simulink model "c_citation"  (R2020a)
settings: Solver=ode5  StartTime=0.0  StopTime=inf  FixedStep=0.01  RelTol=1e-3
InitFcn:
  | load('simulation_parameters');
values from neighbouring files (symbols this model uses):
  chord = 1.991    [citdata.mat]
  cv1 = 20000    [gear_params.m]
  cv2 = cv1    (= 20000)    [gear_params.m]
  cv3 = 4000    [gear_params.m]
  cv4 = 20000    [gear_params.m]
  deltagmax1 = 0.25    [gear_params.m]
  deltagmax2 = deltagmax1    (= 0.25)    [gear_params.m]
  deltagmax3 = 0.24    [gear_params.m]
  deltagmax4 = 0.02    [gear_params.m]
  ealphag = [0  0.2618  0.6981; 1  1.3  0.8]    [citdata.mat]
  ealphas = [0  0.2618  0.6981; 0.157  0.157  0.175]    [citdata.mat]
  g0 = 9.80665    [ac_genrl.mat]
  hDME = 0    [ac_genrl.mat]
  hGS = 0    [ac_genrl.mat]
  kt1 = 525020    [gear_params.m]
  kt2 = kt1    (= 525020)    [gear_params.m]
  kt3 = 457050    [gear_params.m]
  lh = 5.53    [citdata.mat]
  matbuaf = [0  -0.1745  0.4363; 0  -0.1  -0.1; 0.6981  -0.1  -0.1]    [citdata.mat]
  matdaf = [0 0 0.2618 0.6981 0.734842105263 0.771584210526 0.808326315789 0.845068421053 0.881810526316 0.918552631579 0.955294736842 0.992036842105 ... (529 elements, 23x23)]    [citdata.mat]
  matdam = [0 0.05 0.15 0.25 0.35 0.45 0.55 0.65 0.75 0.803571428571 0.857142857143 0.910714285714 ... (529 elements, 23x23)]    [citdata.mat]
  matdbbf = [0 0 0.6981 0.74464 0.79118 0.83772 0.88426 0.9308 0.97734 1.02388 1.07042 1.11696 ... (324 elements, 18x18)]    [citdata.mat]
  matdeaf = [0 0 0.2618 0.6981 0.734842105263 0.771584210526 0.808326315789 0.845068421053 0.881810526316 0.918552631579 0.955294736842 0.992036842105 ... (529 elements, 23x23)]    [citdata.mat]
  matdgaf = [0 0 0.2618 0.6981 -0.1745 -0.0175 -0.008 -0.009 0.4363 -0.0175 -0.008 -0.009 ... (16 elements, 4x4)]    [citdata.mat]
  matdqaf = [0 0 0.2618 0.6981 0.734842105263 0.771584210526 0.808326315789 0.845068421053 0.881810526316 0.918552631579 0.955294736842 0.992036842105 ... (529 elements, 23x23)]    [citdata.mat]
  matduaf = [0 0 0.2618 0.6981 0.734842105263 0.771584210526 0.808326315789 0.845068421053 0.881810526316 0.918552631579 0.955294736842 0.992036842105 ... (529 elements, 23x23)]    [citdata.mat]
  matdwaw = [0 0 0.1745 0.3491 0.5236 0.6458 1.2916 -0.1745 0 0.0018 0.0046 0.0088 ... (49 elements, 7x7)]    [citdata.mat]
  matedhr = [0 1 1 0.71 2 0.51 3 0.34 5 0.12 7.5 0.03 ... (20 elements, 2x10)]    [citdata.mat]
  mateif = [0  0.2618  0.6981; 0  -0.075  -0.075]    [citdata.mat]
  matelhr = [0 1 1 0.95 2 0.91 3 0.84 5 0.71 7.5 0.35 ... (20 elements, 2x10)]    [citdata.mat]
  matemhr = [0 1 1 0.9 2 0.8 3 0.7 5 0.5 7.5 0.25 ... (20 elements, 2x10)]    [citdata.mat]
  matemv1 = [0  90  100; 0  1  1]    [citdata.mat]
  matemv2 = [20  75  90; 0  1  1]    [citdata.mat]
  matemve = [0  90  100; 0  1  1]    [citdata.mat]
  matetam = [0  -0.1745  0.4363; 0  -0.04  -0.04; 1  -0.04  -0.04]    [citdata.mat]
  mateuaf = [0 0 0.6981 0.733005 0.76791 0.802815 0.83772 0.872625 0.90753 0.942435 0.97734 1.012245 ... (529 elements, 23x23)]    [citdata.mat]
  matfaaf = [0 0 0.2618 0.6981 0.734842105263 0.771584210526 0.808326315789 0.845068421053 0.881810526316 0.918552631579 0.955294736842 0.992036842105 ... (529 elements, 23x23)]    [citdata.mat]
  matfaxl = [0.15  0.35; 1  1]    [citdata.mat]
  matibaf = [0 0 0.2618 0.6981 -0.2 -0.119 -0.117 -0.108 0.3 -0.059 -0.052 -0.038 ... (16 elements, 4x4)]    [citdata.mat]
  matibb = [0 0 0.2618 1.571 3.142 -0.2 0 0 0.074 0.124 0 0 ... (50 elements, 5x10)]    [citdata.mat]
  matibmh = [0 0 15000 17142.8571429 19285.7142857 21428.5714286 23571.4285714 25714.2857143 27857.1428571 30000 0 0 ... (100 elements, 10x10)]    [citdata.mat]
  matipaf = [0  -0.1745  0.4363; 0  -0.44  -0.44; 0.6981  -0.44  -0.44]    [citdata.mat]
  matipmh = [0 0 15000 17142.8571429 19285.7142857 21428.5714286 23571.4285714 25714.2857143 27857.1428571 30000 0 0 ... (100 elements, 10x10)]    [citdata.mat]
  matiraf = [0 0 0.2618 0.6981 -0.2 0.05 -0.03 0.01 0.3 0.3 0.37 0.41 ... (16 elements, 4x4)]    [citdata.mat]
  matiuaf = [0  -0.2  0.3; 0  0.052  -0.003; 0.6981  0.052  -0.003]    [citdata.mat]
  matiwaf = [0  -0.1745  0.4363; 0  -0.185  -0.185; 0.6981  -0.185  -0.185]    [citdata.mat]
  matlaf = [0 0 0.2618 0.6981 0.734842105263 0.771584210526 0.808326315789 0.845068421053 0.881810526316 0.918552631579 0.955294736842 0.992036842105 ... (529 elements, 23x23)]    [citdata.mat]
  matlam = [0 0.05 0.15 0.25 0.35 0.45 0.55 0.65 0.75 0.803571428571 0.857142857143 0.910714285714 ... (529 elements, 23x23)]    [citdata.mat]
  matleaf = [0 0 0.2618 0.6981 0.734842105263 0.771584210526 0.808326315789 0.845068421053 0.881810526316 0.918552631579 0.955294736842 0.992036842105 ... (529 elements, 23x23)]    [citdata.mat]
  matleam = [0  -0.1745  0.4363; 0  0.58  0.58; 1  0.58  0.58]    [citdata.mat]
  matlgaf = [0 0 0.2618 0.6981 -0.1745 0.045 0.105 0.14 0.4363 0.045 0.105 0.14 ... (16 elements, 4x4)]    [citdata.mat]
  matlqaf = [0 0 0.2618 0.6981 0.734842105263 0.771584210526 0.808326315789 0.845068421053 0.881810526316 0.918552631579 0.955294736842 0.992036842105 ... (529 elements, 23x23)]    [citdata.mat]
  matluaf = [0 0 0.2618 0.6981 0.734842105263 0.771584210526 0.808326315789 0.845068421053 0.881810526316 0.918552631579 0.955294736842 0.992036842105 ... (529 elements, 23x23)]    [citdata.mat]
  matmaaf = [0 0 0.2618 0.6981 0.734842105263 0.771584210526 0.808326315789 0.845068421053 0.881810526316 0.918552631579 0.955294736842 0.992036842105 ... (484 elements, 22x22)]    [citdata.mat]
  matmaam = [0 0.05 0.15 0.25 0.35 0.45 0.55 0.65 0.75 0.803571428571 0.857142857143 0.910714285714 ... (484 elements, 22x22)]    [citdata.mat]
  matmaf = [0 0 0.2618 0.6981 0.734842105263 0.771584210526 0.808326315789 0.845068421053 0.881810526316 0.918552631579 0.955294736842 0.992036842105 ... (529 elements, 23x23)]    [citdata.mat]
  matmam = [0 0.05 0.15 0.25 0.35 0.45 0.55 0.65 0.75 0.803571428571 0.857142857143 0.910714285714 ... (529 elements, 23x23)]    [citdata.mat]
  matmbbf = [0 0 0.6981 0.74464 0.79118 0.83772 0.88426 0.9308 0.97734 1.02388 1.07042 1.11696 ... (324 elements, 18x18)]    [citdata.mat]
  matmeaf = [0 0 0.2618 0.6981 0.734842105263 0.771584210526 0.808326315789 0.845068421053 0.881810526316 0.918552631579 0.955294736842 0.992036842105 ... (529 elements, 23x23)]    [citdata.mat]
  matmeam = [0 0 1 1.05 1.1 1.15 1.2 1.25 1.3 1.35 1.4 1.45 ... (529 elements, 23x23)]    [citdata.mat]
  matmgaf = [0 0 0.2618 0.6981 -0.1745 -0.01 -0.024 -0.035 0.4363 -0.01 -0.024 -0.035 ... (16 elements, 4x4)]    [citdata.mat]
  matmqaf = [0 0 0.2618 0.6981 0.734842105263 0.771584210526 0.808326315789 0.845068421053 0.881810526316 0.918552631579 0.955294736842 0.992036842105 ... (529 elements, 23x23)]    [citdata.mat]
  matmrbr = [0  0  0.5236; 0  0  0; 0.384  0.001  0.001]    [citdata.mat]
  matnbab = [0 0 0.2618 1.571 3.142 -0.2 0 0 -0.0199 -0.1049 0 0 ... (25 elements, 5x5)]    [citdata.mat]
  matnbaf = [0  -0.2  0.3; 0  0.105  0.18; 0.6981  0.105  0.18]    [citdata.mat]
  matnbmh = [0 0 15000 17142.8571429 19285.7142857 21428.5714286 23571.4285714 25714.2857143 27857.1428571 30000 0 0 ... (100 elements, 10x10)]    [citdata.mat]
  matnpaf = [0 0 0.2618 0.6981 -0.2 0.03 0.03 0.05 0.3 -0.12 -0.12 -0.2 ... (16 elements, 4x4)]    [citdata.mat]
  matnpmh = [0 0 15000 17142.8571429 19285.7142857 21428.5714286 23571.4285714 25714.2857143 27857.1428571 30000 0 0 ... (100 elements, 10x10)]    [citdata.mat]
  matnraf = [0  -0.1745  0.4363; 0  -0.21  -0.21; 0.6981  -0.21  -0.21]    [citdata.mat]
  matnuaf = [0  -0.1745  0.4363; 0  -0.101  -0.101; 0.6981  -0.101  -0.101]    [citdata.mat]
  matnwaf = [0 0 0.2618 0.6981 -0.2 -0.02 -0.037 -0.049 0.3 0.03 0.043 0.036 ... (16 elements, 4x4)]    [citdata.mat]
  matnwmh = [0 0 15000 17142.8571429 19285.7142857 21428.5714286 23571.4285714 25714.2857143 27857.1428571 30000 0 0 ... (100 elements, 10x10)]    [citdata.mat]
  matqlaf = [0  -0.1745  0.4363; 0  -1  -1; 0.6981  -1  -1]    [citdata.mat]
  matquaf = [0 0 0.6981 0.733005 0.76791 0.802815 0.83772 0.872625 0.90753 0.942435 0.97734 1.012245 ... (529 elements, 23x23)]    [citdata.mat]
  matqxl = [0.15  0.35; 1  1]    [citdata.mat]
  matqxm = [0.15  0.35; 1  1]    [citdata.mat]
  matrtam = [0  -0.1745  0.4363; 0  0.011  0.011; 1  0.011  0.011]    [citdata.mat]
  matruaf = [0  -0.1745  0.4363; 0  0.2  0.2; 0.6981  0.2  0.2]    [citdata.mat]
  matrumh = [0 0 15000 17142.8571429 19285.7142857 21428.5714286 23571.4285714 25714.2857143 27857.1428571 30000 0 0 ... (100 elements, 10x10)]    [citdata.mat]
  matuut = [0  0.5  1; 0  1.35  1]    [citdata.mat]
  matwtam = [0  -0.1745  0.4363; 0  0.011  0.011; 1  0.011  0.011]    [citdata.mat]
  matybab = [0 0 0.2618 1.571 3.142 -0.2 0 0 0.34 0.75 0 0 ... (25 elements, 5x5)]    [citdata.mat]
  matybaf = [0  -0.1745  0.4363; 0  -0.75  -0.75; 0.6981  -0.75  -0.75]    [citdata.mat]
  matyraf = [0  -0.1745  0.4363; 0  0.85  0.85; 0.6981  0.85  0.85]    [citdata.mat]
  matyuaf = [0  -0.1745  0.4363; 0  0.23  0.23; 0.6981  0.23  0.23]    [citdata.mat]
  matywaf = [0  -0.1745  0.4363; 0  -0.04  -0.04; 0.6981  -0.04  -0.04]    [citdata.mat]
  murol = 0.03*10    (= 0.3)    [gear_params.m]
  P1 = 2000    [gear_params.m]
  P2 = P1    (= 2000)    [gear_params.m]
  P3 = 2550    [gear_params.m]
  P4 = 40000    [gear_params.m]
  psiLOC = 0    [ac_genrl.mat]
  pstat0 = 101325    [ac_genrl.mat]
  S = 24.99    [citdata.mat]
  span = 13.325    [citdata.mat]
  T0 = 288.15    [ac_genrl.mat]
  tilteng = [0 0]    [citdata.mat]
  toweng = [0 0]    [citdata.mat]
  vdommyr37 = [0  0.2618  0.6981; 0  0.025  0]    [citdata.mat]
  vdommyr38 = [0  0.2618  0.6981; -0.01  0  -0.01]    [citdata.mat]
  Vw915 = 0    [initcit.m]
  winddir = 45*(pi/180)    (= 0.785398163397)    [initcit.m]
  xcgref = 6.5    [citdata.mat]
  xDME = 0    [ac_genrl.mat]
  xeng = [8.407 8.407]    [citdata.mat]
  xGS = 0    [ac_genrl.mat]
  xiacc = 3.2    [ac_genrl.mat]
  xl1 = xcg-6.858    [gear_params.m]
  xl2 = xcg-6.858    [gear_params.m]
  xl3 = xcg-2.0752    [gear_params.m]
  xl4 = xcg-12.742    [gear_params.m]
  xLOC = 0    [ac_genrl.mat]
  ycgref = 0    [citdata.mat]
  yDME = 0    [ac_genrl.mat]
  yeng = [3 -3]    [citdata.mat]
  yGS = 0    [ac_genrl.mat]
  yiacc = 0    [ac_genrl.mat]
  yl1 = 1.918    [gear_params.m]
  yl2 = -1.918    [gear_params.m]
  yl3 = 0    [gear_params.m]
  ... (+9 more)
undefined symbols (not defined in the file or in its folder): Deng, massinit, matff, matn1d, matn2d, matthr, u0, ut0, x0, xt0
(part 5 of 5)

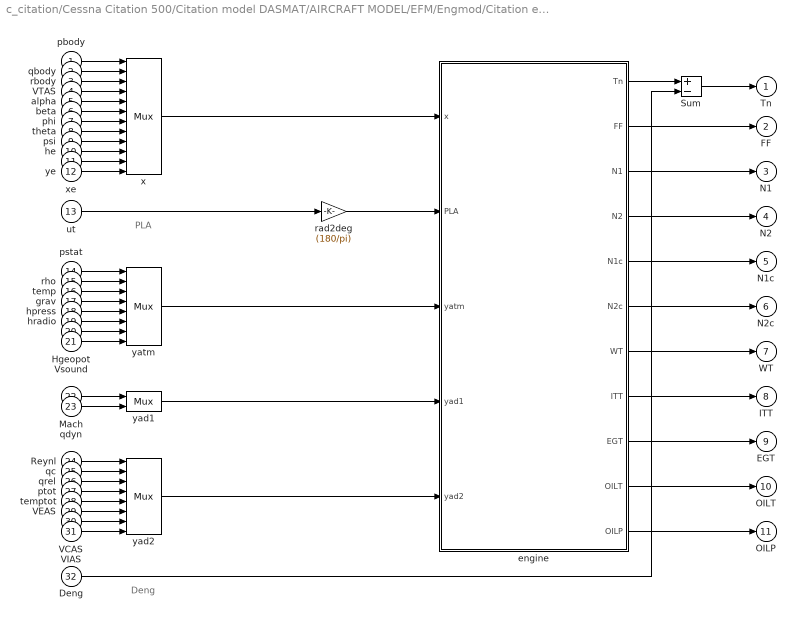
== system c_citation/Cessna Citation 500/Citation model DASMAT/AIRCRAFT MODEL/EFM/Engmod/Citation eng_mod/Subsystem1/JT15 Dynamic1/Subsystem ==
  note: Deng
  note: PLA
  pbody : Inport
  qbody : Inport  Port=2
  rbody : Inport  Port=3
  VTAS : Inport  Port=4
  alpha : Inport  Port=5
  beta : Inport  Port=6
  phi : Inport  Port=7
  theta : Inport  Port=8
  psi : Inport  Port=9
  he : Inport  Port=10
  xe : Inport  Port=11
  ye : Inport  Port=12
  ut : Inport  Port=13
  pstat : Inport  Port=14
  rho : Inport  Port=15
  temp : Inport  Port=16
  grav : Inport  Port=17
  hpress : Inport  Port=18
  hradio : Inport  Port=19
  Hgeopot : Inport  Port=20
  Vsound : Inport  Port=21
  Mach : Inport  Port=22
  qdyn : Inport  Port=23
  Reynl : Inport  Port=24
  qc : Inport  Port=25
  qrel : Inport  Port=26
  ptot : Inport  Port=27
  temptot : Inport  Port=28
  VEAS : Inport  Port=29
  VCAS : Inport  Port=30
  VIAS : Inport  Port=31
  Deng : Inport  Port=32
  Sum : Sum  Inputs=+-  InputSameDT=on  SaturateOnIntegerOverflow=on  OutDataTypeStr=Inherit: Same as first input
  engine : Subsystem
  rad2deg : Gain  Gain=(180/pi)  SaturateOnIntegerOverflow=on  OutDataTypeStr=Inherit: Same as input  ParamDataTypeStr=Inherit: Same as input
  x : Mux  Inputs=12
  yad1 : Mux  Inputs=2
  yad2 : Mux  Inputs=8
  yatm : Mux  Inputs=8
  Tn : Outport  VectorParamsAs1DForOutWhenUnconnected=off
  FF : Outport  Port=2  VectorParamsAs1DForOutWhenUnconnected=off
  N1 : Outport  Port=3  VectorParamsAs1DForOutWhenUnconnected=off
  N2 : Outport  Port=4  VectorParamsAs1DForOutWhenUnconnected=off
  N1c : Outport  Port=5  VectorParamsAs1DForOutWhenUnconnected=off
  N2c : Outport  Port=6  VectorParamsAs1DForOutWhenUnconnected=off
  WT : Outport  Port=7  VectorParamsAs1DForOutWhenUnconnected=off
  ITT : Outport  Port=8  VectorParamsAs1DForOutWhenUnconnected=off
  EGT : Outport  Port=9  VectorParamsAs1DForOutWhenUnconnected=off
  OILT : Outport  Port=10  VectorParamsAs1DForOutWhenUnconnected=off
  OILP : Outport  Port=11  VectorParamsAs1DForOutWhenUnconnected=off
  wires:
  Deng/1 -> Sum/2
  engine/1(Tn) -> Sum/1
  Sum/1 -> Tn/1
  Vsound/1 -> yatm/8
  engine/11(OILP) -> OILP/1
  engine/10(OILT) -> OILT/1
  rad2deg/1 -> engine/2(PLA)
  ut/1 -> rad2deg/1
  engine/9(EGT) -> EGT/1
  engine/8(ITT) -> ITT/1
  engine/7(WT) -> WT/1
  engine/6(N2c) -> N2c/1
  engine/5(N1c) -> N1c/1
  engine/4(N2) -> N2/1
  engine/3(N1) -> N1/1
  engine/2(FF) -> FF/1
  yad1/1 -> engine/4(yad1)
  yatm/1 -> engine/3(yatm)
  yad2/1 -> engine/5(yad2)
  qdyn/1 -> yad1/2
  Mach/1 -> yad1/1
  Reynl/1 -> yad2/1
  qc/1 -> yad2/2
  VCAS/1 -> yad2/7
  temptot/1 -> yad2/5
  qrel/1 -> yad2/3
  VIAS/1 -> yad2/8
  VEAS/1 -> yad2/6
  ptot/1 -> yad2/4
  ye/1 -> x/12
  xe/1 -> x/11
  he/1 -> x/10
  psi/1 -> x/9
  VTAS/1 -> x/4
  beta/1 -> x/6
  theta/1 -> x/8
  rbody/1 -> x/3
  alpha/1 -> x/5
  phi/1 -> x/7
  qbody/1 -> x/2
  pbody/1 -> x/1
  pstat/1 -> yatm/1
  rho/1 -> yatm/2
  Hgeopot/1 -> yatm/7
  hpress/1 -> yatm/5
  temp/1 -> yatm/3
  hradio/1 -> yatm/6
  grav/1 -> yatm/4
  x/1 -> engine/1(x)

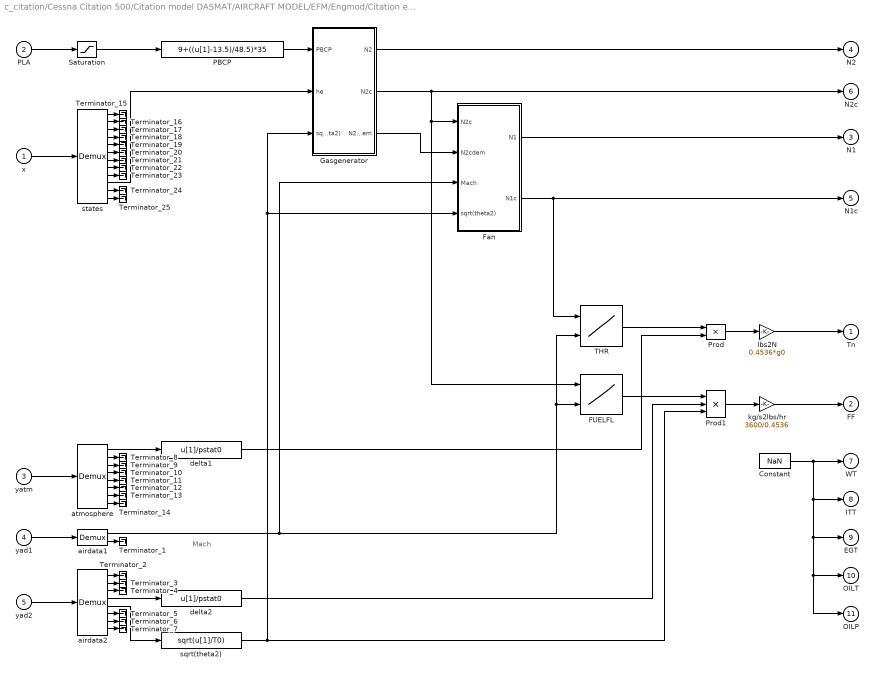
== system c_citation/Cessna Citation 500/Citation model DASMAT/AIRCRAFT MODEL/EFM/Engmod/Citation eng_mod/Subsystem1/JT15 Dynamic/Subsystem/engine ==
  note: Mach
  x : Inport
  PLA : Inport  Port=2
  yatm : Inport  Port=3
  yad1 : Inport  Port=4
  yad2 : Inport  Port=5
  Constant : Constant  Value=NaN
  FUELFL : Lookup2D  RowIndex=matff(2:14,1)  ColumnIndex=matff(1,2:14)  Table=matff(2:14,2:14)  SaturateOnIntegerOverflow=on  InputSameDT=on
  Fan : Subsystem
  Gasgenerator : Subsystem
  PBCP : Fcn  Expr=9+((u[1]-13.5)/48.5)*35
  Prod : Product  InputSameDT=on  SaturateOnIntegerOverflow=on  OutDataTypeStr=Inherit: Same as first input
  Prod1 : Product  Inputs=3  InputSameDT=on  SaturateOnIntegerOverflow=on  OutDataTypeStr=Inherit: Same as first input
  Saturation : Saturate  UpperLimit=62  LowerLimit=13.5
  THR : Lookup2D  RowIndex=matthr(2:12,1)  ColumnIndex=matthr(1,2:12)  Table=matthr(2:12,2:12)  SaturateOnIntegerOverflow=on  InputSameDT=on
  Terminator_{1..25} (25 alike) : Terminator
  airdata1 : Demux  Outputs=2
      settings: DisplayOption=none
  airdata2 : Demux  Outputs=8
      settings: DisplayOption=none
  atmosphere : Demux  Outputs=8
      settings: DisplayOption=none
  delta1 : Fcn  Expr=u[1]/pstat0
  delta2 : Fcn  Expr=u[1]/pstat0
  kg/s2lbs/hr : Gain  Gain=3600/0.4536  SaturateOnIntegerOverflow=on  OutDataTypeStr=Inherit: Same as input  ParamDataTypeStr=Inherit: Same as input
  lbs2N : Gain  Gain=0.4536*g0  SaturateOnIntegerOverflow=on  OutDataTypeStr=Inherit: Same as input  ParamDataTypeStr=Inherit: Same as input
  sqrt(theta2) : Fcn  Expr=sqrt(u[1]/T0)
  states : Demux  Outputs=12
      settings: DisplayOption=none
  Tn : Outport  VectorParamsAs1DForOutWhenUnconnected=off
  FF : Outport  Port=2  VectorParamsAs1DForOutWhenUnconnected=off
  N1 : Outport  Port=3  VectorParamsAs1DForOutWhenUnconnected=off
  N2 : Outport  Port=4  VectorParamsAs1DForOutWhenUnconnected=off
  N1c : Outport  Port=5  VectorParamsAs1DForOutWhenUnconnected=off
  N2c : Outport  Port=6  VectorParamsAs1DForOutWhenUnconnected=off
  WT : Outport  Port=7  VectorParamsAs1DForOutWhenUnconnected=off
  ITT : Outport  Port=8  VectorParamsAs1DForOutWhenUnconnected=off
  EGT : Outport  Port=9  VectorParamsAs1DForOutWhenUnconnected=off
  OILT : Outport  Port=10  VectorParamsAs1DForOutWhenUnconnected=off
  OILP : Outport  Port=11  VectorParamsAs1DForOutWhenUnconnected=off
  wires:
  states/12 -> Terminator_25/1
  states/11 -> Terminator_24/1
  states/9 -> Terminator_23/1
  states/8 -> Terminator_22/1
  states/7 -> Terminator_21/1
  states/6 -> Terminator_20/1
  states/5 -> Terminator_19/1
  states/4 -> Terminator_18/1
  states/3 -> Terminator_17/1
  states/2 -> Terminator_16/1
  states/1 -> Terminator_15/1
  atmosphere/8 -> Terminator_14/1
  atmosphere/7 -> Terminator_13/1
  atmosphere/6 -> Terminator_12/1
  atmosphere/5 -> Terminator_11/1
  atmosphere/4 -> Terminator_10/1
  atmosphere/3 -> Terminator_9/1
  atmosphere/2 -> Terminator_8/1
  airdata2/8 -> Terminator_7/1
  airdata2/7 -> Terminator_6/1
  airdata2/6 -> Terminator_5/1
  airdata2/3 -> Terminator_4/1
  airdata2/2 -> Terminator_3/1
  airdata2/1 -> Terminator_2/1
  airdata1/2 -> Terminator_1/1
  Fan/2(N1c) -> THR/1, N1c/1
  Gasgenerator/2(N2c) -> Fan/1(N2c), FUELFL/1, N2c/1
  Gasgenerator/3(N2cdem) -> Fan/2(N2cdem)
  airdata1/1 -> Fan/3(Mach), FUELFL/2, THR/2
  Fan/1(N1) -> N1/1
  sqrt(theta2)/1 -> Fan/4(sqrt(theta2)), Gasgenerator/3(sqrt(theta2)), Prod1/3
  yad2/1 -> airdata2/1
  yad1/1 -> airdata1/1
  yatm/1 -> atmosphere/1
  airdata2/4 -> delta2/1
  airdata2/5 -> sqrt(theta2)/1
  Constant/1 -> ITT/1, EGT/1, OILT/1, OILP/1, WT/1
  Gasgenerator/1(N2) -> N2/1
  delta1/1 -> Prod/2
  Prod/1 -> lbs2N/1
  THR/1 -> Prod/1
  lbs2N/1 -> Tn/1
  states/10 -> Gasgenerator/2(he)
  delta2/1 -> Prod1/2
  atmosphere/1 -> delta1/1
  Prod1/1 -> kg/s2lbs/hr/1
  kg/s2lbs/hr/1 -> FF/1
  Saturation/1 -> PBCP/1
  PLA/1 -> Saturation/1
  x/1 -> states/1
  PBCP/1 -> Gasgenerator/1(PBCP)
  FUELFL/1 -> Prod1/1

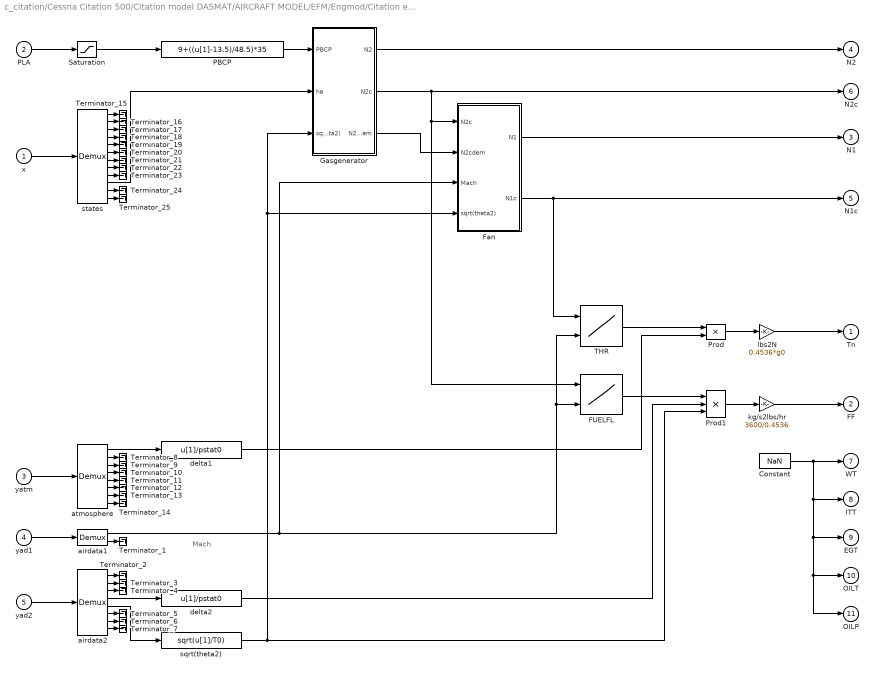
== system c_citation/Cessna Citation 500/Citation model DASMAT/AIRCRAFT MODEL/EFM/Engmod/Citation eng_mod/Subsystem1/JT15 Dynamic1/Subsystem/engine ==
  note: Mach
  x : Inport
  PLA : Inport  Port=2
  yatm : Inport  Port=3
  yad1 : Inport  Port=4
  yad2 : Inport  Port=5
  Constant : Constant  Value=NaN
  FUELFL : Lookup2D  RowIndex=matff(2:14,1)  ColumnIndex=matff(1,2:14)  Table=matff(2:14,2:14)  SaturateOnIntegerOverflow=on  InputSameDT=on
  Fan : Subsystem
  Gasgenerator : Subsystem
  PBCP : Fcn  Expr=9+((u[1]-13.5)/48.5)*35
  Prod : Product  InputSameDT=on  SaturateOnIntegerOverflow=on  OutDataTypeStr=Inherit: Same as first input
  Prod1 : Product  Inputs=3  InputSameDT=on  SaturateOnIntegerOverflow=on  OutDataTypeStr=Inherit: Same as first input
  Saturation : Saturate  UpperLimit=62  LowerLimit=13.5
  THR : Lookup2D  RowIndex=matthr(2:12,1)  ColumnIndex=matthr(1,2:12)  Table=matthr(2:12,2:12)  SaturateOnIntegerOverflow=on  InputSameDT=on
  Terminator_{1..25} (25 alike) : Terminator
  airdata1 : Demux  Outputs=2
      settings: DisplayOption=none
  airdata2 : Demux  Outputs=8
      settings: DisplayOption=none
  atmosphere : Demux  Outputs=8
      settings: DisplayOption=none
  delta1 : Fcn  Expr=u[1]/pstat0
  delta2 : Fcn  Expr=u[1]/pstat0
  kg/s2lbs/hr : Gain  Gain=3600/0.4536  SaturateOnIntegerOverflow=on  OutDataTypeStr=Inherit: Same as input  ParamDataTypeStr=Inherit: Same as input
  lbs2N : Gain  Gain=0.4536*g0  SaturateOnIntegerOverflow=on  OutDataTypeStr=Inherit: Same as input  ParamDataTypeStr=Inherit: Same as input
  sqrt(theta2) : Fcn  Expr=sqrt(u[1]/T0)
  states : Demux  Outputs=12
      settings: DisplayOption=none
  Tn : Outport  VectorParamsAs1DForOutWhenUnconnected=off
  FF : Outport  Port=2  VectorParamsAs1DForOutWhenUnconnected=off
  N1 : Outport  Port=3  VectorParamsAs1DForOutWhenUnconnected=off
  N2 : Outport  Port=4  VectorParamsAs1DForOutWhenUnconnected=off
  N1c : Outport  Port=5  VectorParamsAs1DForOutWhenUnconnected=off
  N2c : Outport  Port=6  VectorParamsAs1DForOutWhenUnconnected=off
  WT : Outport  Port=7  VectorParamsAs1DForOutWhenUnconnected=off
  ITT : Outport  Port=8  VectorParamsAs1DForOutWhenUnconnected=off
  EGT : Outport  Port=9  VectorParamsAs1DForOutWhenUnconnected=off
  OILT : Outport  Port=10  VectorParamsAs1DForOutWhenUnconnected=off
  OILP : Outport  Port=11  VectorParamsAs1DForOutWhenUnconnected=off
  wires:
  states/12 -> Terminator_25/1
  states/11 -> Terminator_24/1
  states/9 -> Terminator_23/1
  states/8 -> Terminator_22/1
  states/7 -> Terminator_21/1
  states/6 -> Terminator_20/1
  states/5 -> Terminator_19/1
  states/4 -> Terminator_18/1
  states/3 -> Terminator_17/1
  states/2 -> Terminator_16/1
  states/1 -> Terminator_15/1
  atmosphere/8 -> Terminator_14/1
  atmosphere/7 -> Terminator_13/1
  atmosphere/6 -> Terminator_12/1
  atmosphere/5 -> Terminator_11/1
  atmosphere/4 -> Terminator_10/1
  atmosphere/3 -> Terminator_9/1
  atmosphere/2 -> Terminator_8/1
  airdata2/8 -> Terminator_7/1
  airdata2/7 -> Terminator_6/1
  airdata2/6 -> Terminator_5/1
  airdata2/3 -> Terminator_4/1
  airdata2/2 -> Terminator_3/1
  airdata2/1 -> Terminator_2/1
  airdata1/2 -> Terminator_1/1
  Fan/2(N1c) -> THR/1, N1c/1
  Gasgenerator/2(N2c) -> Fan/1(N2c), FUELFL/1, N2c/1
  Gasgenerator/3(N2cdem) -> Fan/2(N2cdem)
  airdata1/1 -> Fan/3(Mach), FUELFL/2, THR/2
  Fan/1(N1) -> N1/1
  sqrt(theta2)/1 -> Fan/4(sqrt(theta2)), Gasgenerator/3(sqrt(theta2)), Prod1/3
  yad2/1 -> airdata2/1
  yad1/1 -> airdata1/1
  yatm/1 -> atmosphere/1
  airdata2/4 -> delta2/1
  airdata2/5 -> sqrt(theta2)/1
  Constant/1 -> ITT/1, EGT/1, OILT/1, OILP/1, WT/1
  Gasgenerator/1(N2) -> N2/1
  delta1/1 -> Prod/2
  Prod/1 -> lbs2N/1
  THR/1 -> Prod/1
  lbs2N/1 -> Tn/1
  states/10 -> Gasgenerator/2(he)
  delta2/1 -> Prod1/2
  atmosphere/1 -> delta1/1
  Prod1/1 -> kg/s2lbs/hr/1
  kg/s2lbs/hr/1 -> FF/1
  Saturation/1 -> PBCP/1
  PLA/1 -> Saturation/1
  x/1 -> states/1
  PBCP/1 -> Gasgenerator/1(PBCP)
  FUELFL/1 -> Prod1/1

== system c_citation/Cessna Citation 500/Citation model DASMAT/AIRCRAFT MODEL/EFM/Engmod/Citation eng_mod/Subsystem1/JT15 Dynamic/Subsystem/engine/Fan ==
  note: N1c feedback
  note: N1cdot
  N2c : Inport
  N2cdem : Inport  Port=2
  Mach : Inport  Port=3
  sqrt(theta2) : Inport  Port=4
  Droop : Gain  Gain=2  SaturateOnIntegerOverflow=on  OutDataTypeStr=Inherit: Same as input  ParamDataTypeStr=Inherit: Same as input
  Max accel : Subsystem  mask(Min Value){}
      mask help:
      | Output is minimum value of inputs.
      | y=min(u1,u2)
      mask Help: The Min block produces as output the minimum value of two scalars or vectors. If the inputs are vectors, the output will be a vector containing the minimum elements of the vectors.
      mask Display: disp('Min')
  Max decel : Subsystem  mask(Max Value){}
      mask help:
      | Output is maximum value of inputs.
      | y=max(u1,u2)
      mask Help: The Max block produces as output the maximum value of two scalars or vectors. If the inputs are vectors, the output will be a vector containing the maximum elements of the vectors.
      mask Display: disp('Max')
  N1 state : Integrator  InitialCondition=xt0(2)
  N1D : Lookup2D  RowIndex=matn1d(2:14,1)  ColumnIndex=matn1d(1,2:14)  Table=matn1d(2:14,2:14)  SaturateOnIntegerOverflow=on  InputSameDT=on
  Prod : Product  InputSameDT=on  SaturateOnIntegerOverflow=on  OutDataTypeStr=Inherit: Same as first input
  Sum : Sum  Inputs=+-  InputSameDT=on  SaturateOnIntegerOverflow=on  OutDataTypeStr=Inherit: Same as first input
  fN1cmax : Lookup  InputValues="[0 25 40 70 94  120]"  Table="[0   0   1   12 14  18]"  SaturateOnIntegerOverflow=on
  fN1cmin : Lookup  InputValues="[25     50   60   94 100]"  Table="[-0.05  -0.05    -1    -30 -28]"  SaturateOnIntegerOverflow=on
  N1 : Outport  VectorParamsAs1DForOutWhenUnconnected=off
  N1c : Outport  Port=2  VectorParamsAs1DForOutWhenUnconnected=off
  wires:
  sqrt(theta2)/1 -> Prod/2
  N1 state/1 -> Prod/1, Sum/2, N1c/1
  N2c/1 -> fN1cmin/1, fN1cmax/1
  Max decel/1(out_1) -> N1 state/1
  N1D/1 -> Sum/1
  Max accel/1(out_1) -> Max decel/1(in_1)
  fN1cmax/1 -> Max accel/2(in_2)
  fN1cmin/1 -> Max decel/2(in_2)
  Sum/1 -> Droop/1
  Droop/1 -> Max accel/1(in_1)
  Mach/1 -> N1D/2
  Prod/1 -> N1/1
  N2cdem/1 -> N1D/1

== system c_citation/Cessna Citation 500/Citation model DASMAT/AIRCRAFT MODEL/EFM/Engmod/Citation eng_mod/Subsystem1/JT15 Dynamic/Subsystem/engine/Gasgenerator ==
  note: N2 feedback
  note: N2dot
  PBCP : Inport
  he : Inport  Port=2
  sqrt(theta2) : Inport  Port=3
  Droop : Lookup  InputValues=[0 100]  Table="[0.1  2]"  SaturateOnIntegerOverflow=on
  Fcn : Fcn  Expr=u[1]/u[2]
  Fcn1 : Fcn  Expr=u[1]/u[2]
  Governor : Product  InputSameDT=on  SaturateOnIntegerOverflow=on  OutDataTypeStr=Inherit: Same as first input
  Max accel : Subsystem  mask(Max Value){}
      mask help:
      | Output is maximum value of inputs.
      | y=max(u1,u2)
      mask Help: The Max block produces as output the maximum value of two scalars or vectors. If the inputs are vectors, the output will be a vector containing the maximum elements of the vectors.
      mask Display: disp('Max')
  Min accel : Subsystem  mask(Min Value){}
      mask help:
      | Output is minimum value of inputs.
      | y=min(u1,u2)
      mask Help: The Min block produces as output the minimum value of two scalars or vectors. If the inputs are vectors, the output will be a vector containing the minimum elements of the vectors.
      mask Display: disp('Min')
  Mux : Mux  Inputs=2
  Mux1 : Mux  Inputs=2
  N2 state : Integrator  InitialCondition=xt0(1)
  N2D : Lookup2D  RowIndex=matn2d(2:10,1)  ColumnIndex=matn2d(1,2:10)  Table=matn2d(2:10,2:10)  SaturateOnIntegerOverflow=on  InputSameDT=on
  Sum : Sum  Inputs=+-  InputSameDT=on  SaturateOnIntegerOverflow=on  OutDataTypeStr=Inherit: Same as first input
  fN2max : Lookup  InputValues=[25 40 70 94]  Table=[0 3 8 10]  SaturateOnIntegerOverflow=on
  fN2min : Lookup  InputValues="[25     50   60   94 100]"  Table="[-0.05  -0.05    -2    -20 -28]"  SaturateOnIntegerOverflow=on
  ft2FL : Gain  Gain=.01  SaturateOnIntegerOverflow=on  OutDataTypeStr=Inherit: Same as input  ParamDataTypeStr=Inherit: Same as input
  m2ft : Gain  Gain=(1/0.3048)  SaturateOnIntegerOverflow=on  OutDataTypeStr=Inherit: Same as input  ParamDataTypeStr=Inherit: Same as input
  N2 : Outport  VectorParamsAs1DForOutWhenUnconnected=off
  N2c : Outport  Port=2  VectorParamsAs1DForOutWhenUnconnected=off
  N2cdem : Outport  Port=3  VectorParamsAs1DForOutWhenUnconnected=off
  wires:
  sqrt(theta2)/1 -> Mux1/2, Mux/2
  N2D/1 -> Mux/1, Droop/1, Sum/1
  Fcn1/1 -> N2c/1
  Fcn/1 -> N2cdem/1
  Mux1/1 -> Fcn1/1
  Mux/1 -> Fcn/1
  Min accel/1(out_1) -> Max accel/1(in_1)
  ft2FL/1 -> N2D/2
  m2ft/1 -> ft2FL/1
  he/1 -> m2ft/1
  N2 state/1 -> Mux1/1, fN2min/1, fN2max/1, Sum/2, N2/1
  fN2max/1 -> Min accel/2(in_2)
  fN2min/1 -> Max accel/2(in_2)
  PBCP/1 -> N2D/1
  Droop/1 -> Governor/1
  Sum/1 -> Governor/2
  Governor/1 -> Min accel/1(in_1)
  Max accel/1(out_1) -> N2 state/1

== system c_citation/Cessna Citation 500/Citation model DASMAT/AIRCRAFT MODEL/EFM/Engmod/Citation eng_mod/Subsystem1/JT15 Dynamic1/Subsystem/engine/Fan ==
  note: N1c feedback
  note: N1cdot
  N2c : Inport
  N2cdem : Inport  Port=2
  Mach : Inport  Port=3
  sqrt(theta2) : Inport  Port=4
  Droop : Gain  Gain=2  SaturateOnIntegerOverflow=on  OutDataTypeStr=Inherit: Same as input  ParamDataTypeStr=Inherit: Same as input
  Max accel : Subsystem  mask(Min Value){}
      mask help:
      | Output is minimum value of inputs.
      | y=min(u1,u2)
      mask Help: The Min block produces as output the minimum value of two scalars or vectors. If the inputs are vectors, the output will be a vector containing the minimum elements of the vectors.
      mask Display: disp('Min')
  Max decel : Subsystem  mask(Max Value){}
      mask help:
      | Output is maximum value of inputs.
      | y=max(u1,u2)
      mask Help: The Max block produces as output the maximum value of two scalars or vectors. If the inputs are vectors, the output will be a vector containing the maximum elements of the vectors.
      mask Display: disp('Max')
  N1 state : Integrator  InitialCondition=xt0(2)
  N1D : Lookup2D  RowIndex=matn1d(2:14,1)  ColumnIndex=matn1d(1,2:14)  Table=matn1d(2:14,2:14)  SaturateOnIntegerOverflow=on  InputSameDT=on
  Prod : Product  InputSameDT=on  SaturateOnIntegerOverflow=on  OutDataTypeStr=Inherit: Same as first input
  Sum : Sum  Inputs=+-  InputSameDT=on  SaturateOnIntegerOverflow=on  OutDataTypeStr=Inherit: Same as first input
  fN1cmax : Lookup  InputValues="[0 25 40 70 94  120]"  Table="[0   0   1   12 14  18]"  SaturateOnIntegerOverflow=on
  fN1cmin : Lookup  InputValues="[25     50   60   94 100]"  Table="[-0.05  -0.05    -1    -30 -28]"  SaturateOnIntegerOverflow=on
  N1 : Outport  VectorParamsAs1DForOutWhenUnconnected=off
  N1c : Outport  Port=2  VectorParamsAs1DForOutWhenUnconnected=off
  wires:
  sqrt(theta2)/1 -> Prod/2
  N1 state/1 -> Prod/1, Sum/2, N1c/1
  N2c/1 -> fN1cmin/1, fN1cmax/1
  Max decel/1(out_1) -> N1 state/1
  N1D/1 -> Sum/1
  Max accel/1(out_1) -> Max decel/1(in_1)
  fN1cmax/1 -> Max accel/2(in_2)
  fN1cmin/1 -> Max decel/2(in_2)
  Sum/1 -> Droop/1
  Droop/1 -> Max accel/1(in_1)
  Mach/1 -> N1D/2
  Prod/1 -> N1/1
  N2cdem/1 -> N1D/1

== system c_citation/Cessna Citation 500/Citation model DASMAT/AIRCRAFT MODEL/EFM/Engmod/Citation eng_mod/Subsystem1/JT15 Dynamic1/Subsystem/engine/Gasgenerator ==
  note: N2 feedback
  note: N2dot
  PBCP : Inport
  he : Inport  Port=2
  sqrt(theta2) : Inport  Port=3
  Droop : Lookup  InputValues=[0 100]  Table="[0.1  2]"  SaturateOnIntegerOverflow=on
  Fcn : Fcn  Expr=u[1]/u[2]
  Fcn1 : Fcn  Expr=u[1]/u[2]
  Governor : Product  InputSameDT=on  SaturateOnIntegerOverflow=on  OutDataTypeStr=Inherit: Same as first input
  Max accel : Subsystem  mask(Max Value){}
      mask help:
      | Output is maximum value of inputs.
      | y=max(u1,u2)
      mask Help: The Max block produces as output the maximum value of two scalars or vectors. If the inputs are vectors, the output will be a vector containing the maximum elements of the vectors.
      mask Display: disp('Max')
  Min accel : Subsystem  mask(Min Value){}
      mask help:
      | Output is minimum value of inputs.
      | y=min(u1,u2)
      mask Help: The Min block produces as output the minimum value of two scalars or vectors. If the inputs are vectors, the output will be a vector containing the minimum elements of the vectors.
      mask Display: disp('Min')
  Mux : Mux  Inputs=2
  Mux1 : Mux  Inputs=2
  N2 state : Integrator  InitialCondition=xt0(1)
  N2D : Lookup2D  RowIndex=matn2d(2:10,1)  ColumnIndex=matn2d(1,2:10)  Table=matn2d(2:10,2:10)  SaturateOnIntegerOverflow=on  InputSameDT=on
  Sum : Sum  Inputs=+-  InputSameDT=on  SaturateOnIntegerOverflow=on  OutDataTypeStr=Inherit: Same as first input
  fN2max : Lookup  InputValues=[25 40 70 94]  Table=[0 3 8 10]  SaturateOnIntegerOverflow=on
  fN2min : Lookup  InputValues="[25     50   60   94 100]"  Table="[-0.05  -0.05    -2    -20 -28]"  SaturateOnIntegerOverflow=on
  ft2FL : Gain  Gain=.01  SaturateOnIntegerOverflow=on  OutDataTypeStr=Inherit: Same as input  ParamDataTypeStr=Inherit: Same as input
  m2ft : Gain  Gain=(1/0.3048)  SaturateOnIntegerOverflow=on  OutDataTypeStr=Inherit: Same as input  ParamDataTypeStr=Inherit: Same as input
  N2 : Outport  VectorParamsAs1DForOutWhenUnconnected=off
  N2c : Outport  Port=2  VectorParamsAs1DForOutWhenUnconnected=off
  N2cdem : Outport  Port=3  VectorParamsAs1DForOutWhenUnconnected=off
  wires:
  sqrt(theta2)/1 -> Mux1/2, Mux/2
  N2D/1 -> Mux/1, Droop/1, Sum/1
  Fcn1/1 -> N2c/1
  Fcn/1 -> N2cdem/1
  Mux1/1 -> Fcn1/1
  Mux/1 -> Fcn/1
  Min accel/1(out_1) -> Max accel/1(in_1)
  ft2FL/1 -> N2D/2
  m2ft/1 -> ft2FL/1
  he/1 -> m2ft/1
  N2 state/1 -> Mux1/1, fN2min/1, fN2max/1, Sum/2, N2/1
  fN2max/1 -> Min accel/2(in_2)
  fN2min/1 -> Max accel/2(in_2)
  PBCP/1 -> N2D/1
  Droop/1 -> Governor/1
  Sum/1 -> Governor/2
  Governor/1 -> Min accel/1(in_1)
  Max accel/1(out_1) -> N2 state/1

== system c_citation/Cessna Citation 500/Citation model DASMAT/AIRCRAFT MODEL/EFM/Engmod/Citation eng_mod/Subsystem1/JT15 Dynamic/Subsystem/engine/Fan/Max accel ==
  in_1 : Inport
  in_2 : Inport  Port=2
  Sum : Sum  Inputs=-+  InputSameDT=on  SaturateOnIntegerOverflow=on  OutDataTypeStr=Inherit: Same as first input
  Switch : Switch  SaturateOnIntegerOverflow=on  InputSameDT=on
  out_1 : Outport  VectorParamsAs1DForOutWhenUnconnected=off
  wires:
  in_1/1 -> Sum/1, Switch/1
  in_2/1 -> Sum/2, Switch/3
  Sum/1 -> Switch/2
  Switch/1 -> out_1/1

== system c_citation/Cessna Citation 500/Citation model DASMAT/AIRCRAFT MODEL/EFM/Engmod/Citation eng_mod/Subsystem1/JT15 Dynamic/Subsystem/engine/Fan/Max decel ==
  in_1 : Inport
  in_2 : Inport  Port=2
  Sum : Sum  Inputs=+-  InputSameDT=on  SaturateOnIntegerOverflow=on  OutDataTypeStr=Inherit: Same as first input
  Switch : Switch  SaturateOnIntegerOverflow=on  InputSameDT=on
  out_1 : Outport  VectorParamsAs1DForOutWhenUnconnected=off
  wires:
  Switch/1 -> out_1/1
  Sum/1 -> Switch/2
  in_2/1 -> Sum/2, Switch/3
  in_1/1 -> Sum/1, Switch/1

== system c_citation/Cessna Citation 500/Citation model DASMAT/AIRCRAFT MODEL/EFM/Engmod/Citation eng_mod/Subsystem1/JT15 Dynamic/Subsystem/engine/Gasgenerator/Max accel ==
  in_1 : Inport
  in_2 : Inport  Port=2
  Sum : Sum  Inputs=+-  InputSameDT=on  SaturateOnIntegerOverflow=on  OutDataTypeStr=Inherit: Same as first input
  Switch : Switch  SaturateOnIntegerOverflow=on  InputSameDT=on
  out_1 : Outport  VectorParamsAs1DForOutWhenUnconnected=off
  wires:
  Switch/1 -> out_1/1
  Sum/1 -> Switch/2
  in_2/1 -> Sum/2, Switch/3
  in_1/1 -> Sum/1, Switch/1

== system c_citation/Cessna Citation 500/Citation model DASMAT/AIRCRAFT MODEL/EFM/Engmod/Citation eng_mod/Subsystem1/JT15 Dynamic/Subsystem/engine/Gasgenerator/Min accel ==
  in_1 : Inport
  in_2 : Inport  Port=2
  Sum : Sum  Inputs=-+  InputSameDT=on  SaturateOnIntegerOverflow=on  OutDataTypeStr=Inherit: Same as first input
  Switch : Switch  SaturateOnIntegerOverflow=on  InputSameDT=on
  out_1 : Outport  VectorParamsAs1DForOutWhenUnconnected=off
  wires:
  in_1/1 -> Sum/1, Switch/1
  in_2/1 -> Sum/2, Switch/3
  Sum/1 -> Switch/2
  Switch/1 -> out_1/1

== system c_citation/Cessna Citation 500/Citation model DASMAT/AIRCRAFT MODEL/EFM/Engmod/Citation eng_mod/Subsystem1/JT15 Dynamic1/Subsystem/engine/Fan/Max accel ==
  in_1 : Inport
  in_2 : Inport  Port=2
  Sum : Sum  Inputs=-+  InputSameDT=on  SaturateOnIntegerOverflow=on  OutDataTypeStr=Inherit: Same as first input
  Switch : Switch  SaturateOnIntegerOverflow=on  InputSameDT=on
  out_1 : Outport  VectorParamsAs1DForOutWhenUnconnected=off
  wires:
  in_1/1 -> Sum/1, Switch/1
  in_2/1 -> Sum/2, Switch/3
  Sum/1 -> Switch/2
  Switch/1 -> out_1/1

== system c_citation/Cessna Citation 500/Citation model DASMAT/AIRCRAFT MODEL/EFM/Engmod/Citation eng_mod/Subsystem1/JT15 Dynamic1/Subsystem/engine/Fan/Max decel ==
  in_1 : Inport
  in_2 : Inport  Port=2
  Sum : Sum  Inputs=+-  InputSameDT=on  SaturateOnIntegerOverflow=on  OutDataTypeStr=Inherit: Same as first input
  Switch : Switch  SaturateOnIntegerOverflow=on  InputSameDT=on
  out_1 : Outport  VectorParamsAs1DForOutWhenUnconnected=off
  wires:
  Switch/1 -> out_1/1
  Sum/1 -> Switch/2
  in_2/1 -> Sum/2, Switch/3
  in_1/1 -> Sum/1, Switch/1

== system c_citation/Cessna Citation 500/Citation model DASMAT/AIRCRAFT MODEL/EFM/Engmod/Citation eng_mod/Subsystem1/JT15 Dynamic1/Subsystem/engine/Gasgenerator/Max accel ==
  in_1 : Inport
  in_2 : Inport  Port=2
  Sum : Sum  Inputs=+-  InputSameDT=on  SaturateOnIntegerOverflow=on  OutDataTypeStr=Inherit: Same as first input
  Switch : Switch  SaturateOnIntegerOverflow=on  InputSameDT=on
  out_1 : Outport  VectorParamsAs1DForOutWhenUnconnected=off
  wires:
  Switch/1 -> out_1/1
  Sum/1 -> Switch/2
  in_2/1 -> Sum/2, Switch/3
  in_1/1 -> Sum/1, Switch/1

== system c_citation/Cessna Citation 500/Citation model DASMAT/AIRCRAFT MODEL/EFM/Engmod/Citation eng_mod/Subsystem1/JT15 Dynamic1/Subsystem/engine/Gasgenerator/Min accel ==
  in_1 : Inport
  in_2 : Inport  Port=2
  Sum : Sum  Inputs=-+  InputSameDT=on  SaturateOnIntegerOverflow=on  OutDataTypeStr=Inherit: Same as first input
  Switch : Switch  SaturateOnIntegerOverflow=on  InputSameDT=on
  out_1 : Outport  VectorParamsAs1DForOutWhenUnconnected=off
  wires:
  in_1/1 -> Sum/1, Switch/1
  in_2/1 -> Sum/2, Switch/3
  Sum/1 -> Switch/2
  Switch/1 -> out_1/1
